simulink library "Contact_Forces_Lib"  (R2019b)
settings: Solver=ode45  StartTime=0.0  StopTime=10.0  RelTol=1e-3  EnableMultiTasking=on
undefined symbols (not defined in the file): b_contact, ball, custom_param_1, custom_param_2, Extr_Data_Ring, k_contact, l_cone, length_cylinder, length_tube, mu_kinetic, mu_static, pen_exponent, pen_full_damp_F, rad_s_cone, radius_cylinder, radius_tube, tube, v_thr, X, Y, Z
libraries: nesl_utility x166, sm_lib x109, $bdroot x65, simulink x14, fl_lib x1
(part 8 of 10)

== system Contact_Forces_Lib/2D/Composite Forces/Box to Box Force/BoxF Corners ==
  Circle to Line C1 AC : $bdroot/2D/Circle to Finite Line Force  circle_rad=boxF_contact_rad  line_depth=boxB_h/2  line_length=boxB_l  force_law=Linear  k_contact=k_contact_box2box  b_contact=b_contact_box2box  pen_full_damp_F=pen_full_damp_F_box2box  pen_exponent=pen_exponent_box2box  custom_param_1=1  custom_param_2=1  friction_law=None  mu_kinetic=mu_kinetic_box2box  mu_static=mu_static_box2box  v_thr=v_thr_box2box  vis_on=off  vis_opc_en=0  vis_len_linBz=vis_len_boxBz  vis_len_linBx=vis_len_boxBx  vis_len_cirFz=vis_len_boxFz  vis_len_cirFx=vis_len_boxFx  vis_clr=vis_clr_box2box  vis_opc=vis_opc_box2box
  Circle to Line C1 BD : $bdroot/2D/Circle to Finite Line Force  circle_rad=boxF_contact_rad  line_depth=boxB_l/2  line_length=boxB_h  force_law=Linear  k_contact=k_contact_box2box  b_contact=b_contact_box2box  pen_full_damp_F=pen_full_damp_F_box2box  pen_exponent=pen_exponent_box2box  custom_param_1=1  custom_param_2=1  friction_law=None  mu_kinetic=mu_kinetic_box2box  mu_static=mu_static_box2box  v_thr=v_thr_box2box  vis_on=off  vis_opc_en=0  vis_len_linBz=vis_len_boxBz  vis_len_linBx=vis_len_boxBx  vis_len_cirFz=vis_len_boxFz  vis_len_cirFx=vis_len_boxFx  vis_clr=vis_clr_box2box  vis_opc=vis_opc_box2box
  Circle to Line C2 AC : $bdroot/2D/Circle to Finite Line Force  circle_rad=boxF_contact_rad  line_depth=boxB_h/2  line_length=boxB_l  force_law=Linear  k_contact=k_contact_box2box  b_contact=b_contact_box2box  pen_full_damp_F=pen_full_damp_F_box2box  pen_exponent=pen_exponent_box2box  custom_param_1=1  custom_param_2=1  friction_law=None  mu_kinetic=mu_kinetic_box2box  mu_static=mu_static_box2box  v_thr=v_thr_box2box  vis_on=off  vis_opc_en=0  vis_len_linBz=vis_len_boxBz  vis_len_linBx=vis_len_boxBx  vis_len_cirFz=vis_len_boxFz  vis_len_cirFx=vis_len_boxFx  vis_clr=vis_clr_box2box  vis_opc=vis_opc_box2box
  Circle to Line C2 BD : $bdroot/2D/Circle to Finite Line Force  circle_rad=boxF_contact_rad  line_depth=boxB_l/2  line_length=boxB_h  force_law=Linear  k_contact=k_contact_box2box  b_contact=b_contact_box2box  pen_full_damp_F=pen_full_damp_F_box2box  pen_exponent=pen_exponent_box2box  custom_param_1=1  custom_param_2=1  friction_law=None  mu_kinetic=mu_kinetic_box2box  mu_static=mu_static_box2box  v_thr=v_thr_box2box  vis_on=off  vis_opc_en=0  vis_len_linBz=vis_len_boxBz  vis_len_linBx=vis_len_boxBx  vis_len_cirFz=vis_len_boxFz  vis_len_cirFx=vis_len_boxFx  vis_clr=vis_clr_box2box  vis_opc=vis_opc_box2box
  Circle to Line C3 AC : $bdroot/2D/Circle to Finite Line Force  circle_rad=boxF_contact_rad  line_depth=boxB_h/2  line_length=boxB_l  force_law=Linear  k_contact=k_contact_box2box  b_contact=b_contact_box2box  pen_full_damp_F=pen_full_damp_F_box2box  pen_exponent=pen_exponent_box2box  custom_param_1=1  custom_param_2=1  friction_law=None  mu_kinetic=mu_kinetic_box2box  mu_static=mu_static_box2box  v_thr=v_thr_box2box  vis_on=off  vis_opc_en=0  vis_len_linBz=vis_len_boxBz  vis_len_linBx=vis_len_boxBx  vis_len_cirFz=vis_len_boxFz  vis_len_cirFx=vis_len_boxFx  vis_clr=vis_clr_box2box  vis_opc=vis_opc_box2box
  Circle to Line C3 BD : $bdroot/2D/Circle to Finite Line Force  circle_rad=boxF_contact_rad  line_depth=boxB_l/2  line_length=boxB_h  force_law=Linear  k_contact=k_contact_box2box  b_contact=b_contact_box2box  pen_full_damp_F=pen_full_damp_F_box2box  pen_exponent=pen_exponent_box2box  custom_param_1=1  custom_param_2=1  friction_law=None  mu_kinetic=mu_kinetic_box2box  mu_static=mu_static_box2box  v_thr=v_thr_box2box  vis_on=off  vis_opc_en=0  vis_len_linBz=vis_len_boxBz  vis_len_linBx=vis_len_boxBx  vis_len_cirFz=vis_len_boxFz  vis_len_cirFx=vis_len_boxFx  vis_clr=vis_clr_box2box  vis_opc=vis_opc_box2box
  Circle to Line C4 AC : $bdroot/2D/Circle to Finite Line Force  circle_rad=boxF_contact_rad  line_depth=boxB_h/2  line_length=boxB_l  force_law=Linear  k_contact=k_contact_box2box  b_contact=b_contact_box2box  pen_full_damp_F=pen_full_damp_F_box2box  pen_exponent=pen_exponent_box2box  custom_param_1=1  custom_param_2=1  friction_law=None  mu_kinetic=mu_kinetic_box2box  mu_static=mu_static_box2box  v_thr=v_thr_box2box  vis_on=off  vis_opc_en=0  vis_len_linBz=vis_len_boxBz  vis_len_linBx=vis_len_boxBx  vis_len_cirFz=vis_len_boxFz  vis_len_cirFx=vis_len_boxFx  vis_clr=vis_clr_box2box  vis_opc=vis_opc_box2box
  Circle to Line C4 BD : $bdroot/2D/Circle to Finite Line Force  circle_rad=boxF_contact_rad  line_depth=boxB_l/2  line_length=boxB_h  force_law=Linear  k_contact=k_contact_box2box  b_contact=b_contact_box2box  pen_full_damp_F=pen_full_damp_F_box2box  pen_exponent=pen_exponent_box2box  custom_param_1=1  custom_param_2=1  friction_law=None  mu_kinetic=mu_kinetic_box2box  mu_static=mu_static_box2box  v_thr=v_thr_box2box  vis_on=off  vis_opc_en=0  vis_len_linBz=vis_len_boxBz  vis_len_linBx=vis_len_boxBx  vis_len_cirFz=vis_len_boxFz  vis_len_cirFx=vis_len_boxFx  vis_clr=vis_clr_box2box  vis_opc=vis_opc_box2box
  Forces : Subsystem
  Transform BD : sm_lib/Frames and Transforms/Rigid Transform  TranslationMethod=None  TranslationStandardOffset=0.1  TranslationLengthUnit=m  TranslationStandardAxis=+Y  TranslationCartesianOffset=[0 0 0]  TranslationROffset=0  TranslationROffsetUnits=m  TranslationZOffset=0  TranslationZOffsetUnits=m  TranslationThetaOffset=0  TranslationThetaOffsetUnits=deg  RotationMethod=StandardAxis  RotationAngleUnits=deg  RotationStandardAxis=+Z  RotationAngle=90  RotationArbitraryAxis=[0 0 1]  FollAlignAxisA=+X  BaseAlignAxisA=+Y  FollAlignAxisB=+Y  BaseAlignAxisB=+Z  RotationSequenceAxes=FollowerAxes  RotationSequence=XYX  RotationSequenceAngles=[0 0 0]  RotationSequenceAnglesUnits=deg  RotationMatrix=[1 0 0; 0 1 0; 0 0 1]
  Transform C1 : sm_lib/Frames and Transforms/Rigid Transform  TranslationMethod=Cartesian  TranslationStandardOffset=0.1  TranslationLengthUnit=m  TranslationStandardAxis=+Y  TranslationCartesianOffset=[-(boxF_h/2-boxF_contact_rad) -(boxF_l/2-boxF_contact_rad) 0]  TranslationROffset=0  TranslationROffsetUnits=m  TranslationZOffset=0  TranslationZOffsetUnits=m  TranslationThetaOffset=0  TranslationThetaOffsetUnits=deg  RotationMethod=None  RotationAngleUnits=deg  RotationStandardAxis=+Z  RotationAngle=0  RotationArbitraryAxis=[0 0 1]  FollAlignAxisA=+X  BaseAlignAxisA=+Y  FollAlignAxisB=+Y  BaseAlignAxisB=+Z  RotationSequenceAxes=FollowerAxes  RotationSequence=XYX  RotationSequenceAngles=[0 0 0]  RotationSequenceAnglesUnits=deg  RotationMatrix=[1 0 0; 0 1 0; 0 0 1]
  Transform C2 : sm_lib/Frames and Transforms/Rigid Transform  TranslationMethod=Cartesian  TranslationStandardOffset=0.1  TranslationLengthUnit=m  TranslationStandardAxis=+Y  TranslationCartesianOffset=[-(boxF_h/2-boxF_contact_rad) (boxF_l/2-boxF_contact_rad) 0]  TranslationROffset=0  TranslationROffsetUnits=m  TranslationZOffset=0  TranslationZOffsetUnits=m  TranslationThetaOffset=0  TranslationThetaOffsetUnits=deg  RotationMethod=None  RotationAngleUnits=deg  RotationStandardAxis=+Z  RotationAngle=0  RotationArbitraryAxis=[0 0 1]  FollAlignAxisA=+X  BaseAlignAxisA=+Y  FollAlignAxisB=+Y  BaseAlignAxisB=+Z  RotationSequenceAxes=FollowerAxes  RotationSequence=XYX  RotationSequenceAngles=[0 0 0]  RotationSequenceAnglesUnits=deg  RotationMatrix=[1 0 0; 0 1 0; 0 0 1]
  Transform C3 : sm_lib/Frames and Transforms/Rigid Transform  TranslationMethod=Cartesian  TranslationStandardOffset=0.1  TranslationLengthUnit=m  TranslationStandardAxis=+Y  TranslationCartesianOffset=[(boxF_h/2-boxF_contact_rad) (boxF_l/2-boxF_contact_rad) 0]  TranslationROffset=0  TranslationROffsetUnits=m  TranslationZOffset=0  TranslationZOffsetUnits=m  TranslationThetaOffset=0  TranslationThetaOffsetUnits=deg  RotationMethod=None  RotationAngleUnits=deg  RotationStandardAxis=+Z  RotationAngle=0  RotationArbitraryAxis=[0 0 1]  FollAlignAxisA=+X  BaseAlignAxisA=+Y  FollAlignAxisB=+Y  BaseAlignAxisB=+Z  RotationSequenceAxes=FollowerAxes  RotationSequence=XYX  RotationSequenceAngles=[0 0 0]  RotationSequenceAnglesUnits=deg  RotationMatrix=[1 0 0; 0 1 0; 0 0 1]
  Transform C4 : sm_lib/Frames and Transforms/Rigid Transform  TranslationMethod=Cartesian  TranslationStandardOffset=0.1  TranslationLengthUnit=m  TranslationStandardAxis=+Y  TranslationCartesianOffset=[(boxF_h/2-boxF_contact_rad) -(boxF_l/2-boxF_contact_rad) 0]  TranslationROffset=0  TranslationROffsetUnits=m  TranslationZOffset=0  TranslationZOffsetUnits=m  TranslationThetaOffset=0  TranslationThetaOffsetUnits=deg  RotationMethod=None  RotationAngleUnits=deg  RotationStandardAxis=+Z  RotationAngle=0  RotationArbitraryAxis=[0 0 1]  FollAlignAxisA=+X  BaseAlignAxisA=+Y  FollAlignAxisB=+Y  BaseAlignAxisB=+Z  RotationSequenceAxes=FollowerAxes  RotationSequence=XYX  RotationSequenceAngles=[0 0 0]  RotationSequenceAnglesUnits=deg  RotationMatrix=[1 0 0; 0 1 0; 0 0 1]
  BoxB : PMIOPort  Side=Left
  BoxF : PMIOPort  Port=2  Side=Right
  wires:
  Circle to Line C4 AC/1 -> Forces/7(4AC)
  Circle to Line C1 BD/1 -> Forces/2(1BD)
  Circle to Line C2 AC/1 -> Forces/3(2AC)
  Circle to Line C3 BD/1 -> Forces/6(3BD)
  Circle to Line C4 BD/1 -> Forces/8(4BD)
  Circle to Line C2 BD/1 -> Forces/4(2BD)
  Circle to Line C3 AC/1 -> Forces/5(3AC)
  Circle to Line C1 AC/1 -> Forces/1(1AC)
  connections:
  Circle to Line C1 BD/RConn1 -- Transform BD/RConn1 -- Circle to Line C3 BD/RConn1 -- Circle to Line C4 BD/RConn1 -- Circle to Line C2 BD/RConn1
  Circle to Line C2 AC/LConn1 -- Circle to Line C2 BD/LConn1 -- Transform C2/RConn1
  Circle to Line C3 AC/LConn1 -- Circle to Line C3 BD/LConn1 -- Transform C3/RConn1
  Transform C3/LConn1 -- Transform C4/LConn1 -- Transform C1/LConn1 -- Transform C2/LConn1 -- BoxF/RConn1
  Circle to Line C4 AC/LConn1 -- Circle to Line C4 BD/LConn1 -- Transform C4/RConn1
  Transform BD/LConn1 -- Circle to Line C1 AC/RConn1 -- Circle to Line C2 AC/RConn1 -- Circle to Line C3 AC/RConn1 -- Circle to Line C4 AC/RConn1 -- BoxB/RConn1
  Circle to Line C1 BD/LConn1 -- Circle to Line C1 AC/LConn1 -- Transform C1/RConn1

== system Contact_Forces_Lib/3D/Prototype/Cone in Ring Force/Enable ==
  z : Inport
  R : Inport  Port=2
  Add1 : Sum  Inputs=+-
  Add3 : Sum  Inputs=+-
  Constant1 : Constant  Value=l_cyl/2+lc
  Constant2 : Constant  Value=l_tube/2
  Constant4 : Constant  Value=l_cyl/2
  Constant5 : Constant  Value=l_tube/2
  Logical Operator : Logic  AllPortsSameDT=off  OutDataTypeStr=boolean
  Product : Product
  Product1 : Product
  Relational Operator1 : RelationalOperator  OutDataTypeStr=boolean  ZeroCross=off  RndMeth=Nearest
  Relational Operator2 : RelationalOperator  Operator=<=  OutDataTypeStr=boolean  ZeroCross=off  RndMeth=Nearest
  Selector : Selector  NumberOfDimensions=2  InputPortWidth=3  IndexOptions=Index vector (dialog),Index vector (dialog)  Indices=3,3  OutputSizes=1,1
  Enable : Outport
  wires:
  Constant5/1 -> Relational Operator1/2
  Add3/1 -> Relational Operator1/1
  Relational Operator1/1 -> Logical Operator/1
  Constant2/1 -> Relational Operator2/2
  z/1 -> Add1/1, Add3/1
  Add1/1 -> Relational Operator2/1
  Relational Operator2/1 -> Logical Operator/2
  Logical Operator/1 -> Enable/1
  R/1 -> Selector/1
  Constant4/1 -> Product/1
  Product/1 -> Add3/2
  Selector/1 -> Product1/1, Product/2  "r33"
  Constant1/1 -> Product1/2
  Product1/1 -> Add1/2

== system Contact_Forces_Lib/3D/Prototype/Cone in Ring Force/If Action Subsystem ==
  Action Port : ActionPort
  Constant : Constant  Value=[0 0 0]  SampleTime=0
  F : Outport
  T : Outport  Port=2
  wires:
  Constant/1 -> T/1, F/1

== system Contact_Forces_Lib/3D/Prototype/Cone in Ring Force/Point of Contact calc ==
  note: Xb = r11*r*cos(th) + r12*r*sin(th) +r13*z + Xc;
      | Yb = r21*r*cos(th) + r22*r*sin(th) +r23*z + Yc;
  R : Inport
  x : Inport  Port=2
  y : Inport  Port=3
  z : Inport  Port=4
  Action Port : ActionPort
  Constant1 : Constant  Value=[0:2*pi/n:2*pi]
  Cross Product : Subsystem
  Demux : Demux  Outputs=3
  Demux1 : Demux  Outputs=3
  Demux2 : Demux  Outputs=3
  Force Calc : Subsystem
  Mux : Mux  Inputs=3
  R1 : InportShadow
  Selector : Selector  NumberOfDimensions=2  InputPortWidth=3  IndexOptions=Index vector (dialog),Index vector (dialog)  Indices=1,[1:3]  OutputSizes=1,1
  Selector1 : Selector  NumberOfDimensions=2  InputPortWidth=3  IndexOptions=Index vector (dialog),Index vector (dialog)  Indices=2,[1:3]  OutputSizes=1,1
  Selector2 : Selector  NumberOfDimensions=2  InputPortWidth=3  IndexOptions=Index vector (dialog),Index vector (dialog)  Indices=3,[1:3]  OutputSizes=1,1
  r calc : Subsystem
  x calc : Subsystem
  y calc : Subsystem
  z calc : Subsystem
  F : Outport
  T : Outport  Port=2
  wires:
  R/1 -> Selector2/1, Selector1/1, Selector/1
  Selector/1 -> Demux/1
  Selector1/1 -> Demux1/1
  Selector2/1 -> Demux2/1
  Demux2/1 -> z calc/1(r31)  "r31"
  Demux2/2 -> z calc/2(r32)  "r32"
  Demux2/3 -> z calc/3(r33)  "r33"
  z/1 -> z calc/4(zc)
  Constant1/1 -> Force Calc/5(th), x calc/5(th), y calc/5(th), z calc/5(th)
  Demux/1 -> x calc/1(r11)
  Demux/2 -> x calc/2(r12)
  Demux/3 -> x calc/3(r13)
  x/1 -> x calc/4(xc)
  z calc/1(z) -> Force Calc/4(z), y calc/6(z), x calc/6(z), r calc/1(z)
  Demux1/1 -> y calc/1(r21)
  Demux1/2 -> y calc/2(r22)
  Demux1/3 -> y calc/3(r23)
  y/1 -> y calc/4(yc)
  x calc/1(x) -> Force Calc/1(x)
  y calc/1(y) -> Force Calc/2(y)
  Force Calc/1(Fx) -> Mux/1
  Force Calc/2(Fy) -> Mux/2
  r calc/1(r) -> Force Calc/3(r), x calc/7(r), y calc/7(r)
  Force Calc/3(Fz) -> Mux/3
  Mux/1 -> Cross Product/2(In2), F/1
  Force Calc/4(pc) -> Cross Product/1(In1)
  Cross Product/1(Out1) -> T/1

== system Contact_Forces_Lib/3D/Prototype/Cylinder In Ring Force/Enable ==
  z : Inport
  R : Inport  Port=2
  Abs : Abs  ZeroCross=off
  Add2 : Sum
  Add3 : Sum  Inputs=+-
  Constant2 : Constant  Value=l_tube/2
  Constant3 : Constant  Value=l_cyl/2
  Constant4 : Constant  Value=l_cyl/2
  Constant5 : Constant  Value=l_tube/2
  Logical Operator : Logic  AllPortsSameDT=off  OutDataTypeStr=boolean
  Product : Product
  Product1 : Product
  Relational Operator : RelationalOperator  OutDataTypeStr=boolean  ZeroCross=off  RndMeth=Nearest
  Relational Operator1 : RelationalOperator  Operator=<=  OutDataTypeStr=boolean  ZeroCross=off  RndMeth=Nearest
  Selector : Selector  NumberOfDimensions=2  InputPortWidth=3  IndexOptions=Index vector (dialog),Index vector (dialog)  Indices=3,3  OutputSizes=1,1
  Enable : Outport
  wires:
  z/1 -> Abs/1
  Logical Operator/1 -> Enable/1
  Constant5/1 -> Relational Operator1/2
  Constant2/1 -> Relational Operator/2
  Relational Operator/1 -> Logical Operator/1
  Abs/1 -> Add3/1, Add2/2
  Relational Operator1/1 -> Logical Operator/2
  Add2/1 -> Relational Operator/1
  Add3/1 -> Relational Operator1/1
  R/1 -> Selector/1
  Selector/1 -> Product1/2, Product/1  "r33"
  Product/1 -> Add3/2
  Constant4/1 -> Product/2
  Product1/1 -> Add2/1
  Constant3/1 -> Product1/1

== system Contact_Forces_Lib/3D/Prototype/Cylinder In Ring Force/If Action Subsystem ==
  Action Port : ActionPort
  Constant : Constant  Value=[0 0 0]  SampleTime=0
  F : Outport
  T : Outport  Port=2
  wires:
  Constant/1 -> T/1, F/1

== system Contact_Forces_Lib/3D/Prototype/Cylinder In Ring Force/Point of Contact calc ==
  note: z = (L/2 - r31*r*cos(th) - r32*r*sin(th) - Zc)/r33;
      | Xb = r11*r*cos(th) + r12*r*sin(th) +r13*z + Xc;
      | Yb = r21*r*cos(th) + r22*r*sin(th) +r23*z + Yc;
  R : Inport
  x : Inport  Port=2
  y : Inport  Port=3
  z : Inport  Port=4
  vz : Inport  Port=5
  Action Port : ActionPort
  Constant1 : Constant  Value=[0:2*pi/n:2*pi]
  Cross Product : Subsystem
  Demux : Demux  Outputs=3
  Demux1 : Demux  Outputs=3
  Demux2 : Demux  Outputs=3
  Divide : Product  Inputs=/*  Multiplication=Matrix(*)
  Force Calc : Subsystem
  Mux : Mux  Inputs=3
  R1 : InportShadow
  Selector : Selector  NumberOfDimensions=2  InputPortWidth=3  IndexOptions=Index vector (dialog),Index vector (dialog)  Indices=1,[1:3]  OutputSizes=1,1
  Selector1 : Selector  NumberOfDimensions=2  InputPortWidth=3  IndexOptions=Index vector (dialog),Index vector (dialog)  Indices=2,[1:3]  OutputSizes=1,1
  Selector2 : Selector  NumberOfDimensions=2  InputPortWidth=3  IndexOptions=Index vector (dialog),Index vector (dialog)  Indices=3,[1:3]  OutputSizes=1,1
  x calc : Subsystem
  y calc : Subsystem
  z calc : Subsystem
  F : Outport
  T : Outport  Port=2
  pen : Outport  Port=3
  wires:
  R/1 -> Selector2/1, Selector1/1, Selector/1
  Selector/1 -> Demux/1
  Selector1/1 -> Demux1/1
  Selector2/1 -> Demux2/1
  Demux2/1 -> z calc/1(r31)  "r31"
  Demux2/2 -> z calc/2(r32)  "r32"
  Demux2/3 -> z calc/3(r33)  "r33"
  z/1 -> z calc/4(zc)
  Constant1/1 -> Force Calc/5(th), y calc/5(th), x calc/5(th), z calc/5(th)
  Demux/1 -> x calc/1(r11)
  Demux/2 -> x calc/2(r12)
  Demux/3 -> x calc/3(r13)
  x/1 -> x calc/4(xc)
  z calc/1(z) -> Force Calc/4(z), y calc/6(z), x calc/6(z)
  Demux1/1 -> y calc/1(r21)
  Demux1/2 -> y calc/2(r22)
  Demux1/3 -> y calc/3(r23)
  y/1 -> y calc/4(yc)
  x calc/1(x) -> Force Calc/1(x)
  y calc/1(y) -> Force Calc/2(y)
  R1/1 -> Divide/1
  Force Calc/1(Fx) -> Mux/1
  Force Calc/2(Fy) -> Mux/2
  Mux/1 -> Divide/2
  Divide/1 -> Cross Product/2(In2), F/1
  Force Calc/3(Fz) -> Mux/3
  Force Calc/4(pc) -> Cross Product/1(In1)
  Cross Product/1(Out1) -> T/1
  vz/1 -> Force Calc/3(v)
  Force Calc/5(maxpen) -> pen/1

== system Contact_Forces_Lib/3D/Sphere in Sphere Force/Ff/Check w or v non zero ==
  w : Inport
  v : Inport  Port=2
  Else : Subsystem  TreatAsAtomicUnit=on
  If : If  NumInputs=2  IfExpression=u1 ~= 0 | u2~=0
  mag v : Subsystem
  mag w : Subsystem
  else v is 0 : Outport
  else uv is 0 : Outport  Port=2
  Use SlipVel : Outport  Port=3
  wires:
  Else/2(vuvect) -> else uv is 0/1
  Else/1(vabs) -> else v is 0/1
  If/2 -> Else/Action
  If/1 -> Use SlipVel/1
  mag w/1(mag) -> If/1
  mag v/1(mag) -> If/2
  v/1 -> mag v/1(vect)
  w/1 -> mag w/1(vect)

== system Contact_Forces_Lib/3D/Sphere in Sphere Force/Ff/SlipVel ==
  w : Inport
  v : Inport  Port=2
  dvect : Inport  Port=3
  Action Port : ActionPort
  Add : Sum
  Add1 : Sum  Inputs=+-
  Add2 : Sum  Inputs=+++
  Cross Product : $bdroot/Math/Cross Product
  Demux : Demux  Outputs=3
  Dot Product : DotProduct  InputSameDT=on  OutDataTypeStr=Inherit: Inherit via internal rule
  Fsphere_rad : Gain  Gain=sphF_rad
  Gain : Gain
  If : If  ShowElse=off
  If Action Subsystem : Subsystem  TreatAsAtomicUnit=on
  Math Function : Math  Operator=square  SaturateOnIntegerOverflow=on
  Math Function1 : Math  Operator=square  SaturateOnIntegerOverflow=on
  Math Function2 : Math  Operator=square  SaturateOnIntegerOverflow=on
  Product : Product
  Sqrt : Sqrt  SaturateOnIntegerOverflow=on
  mag : Subsystem
  vabs : Outport  InitialOutput=0
  vuvect : Outport  Port=2  InitialOutput=0
  wires:
  If Action Subsystem/1(Out1) -> vuvect/1
  If/1 -> If Action Subsystem/Action
  Fsphere_rad/1 -> Cross Product/2
  w/1 -> Cross Product/1
  Cross Product/1 -> Add/1
  v/1 -> Add/2
  dvect/1 -> Gain/1
  Add/1 -> Add1/1, Dot Product/1
  Dot Product/1 -> Product/1
  Product/1 -> Add1/2
  Add1/1 -> Demux/1, mag/1(vect), If Action Subsystem/2(In2)
  Demux/1 -> Math Function/1
  Demux/2 -> Math Function1/1
  Demux/3 -> Math Function2/1
  Math Function/1 -> Add2/1
  Math Function1/1 -> Add2/2
  Math Function2/1 -> Add2/3
  Add2/1 -> Sqrt/1
  Sqrt/1 -> vabs/1
  mag/1(mag) -> If/1, If Action Subsystem/1(In1)
  Gain/1 -> Product/2, Dot Product/2, Fsphere_rad/1

== system Contact_Forces_Lib/3D/Sphere in Sphere Force/Ff/mag ==
  vect : Inport
  Add2 : Sum  Inputs=+++
  Demux : Demux  Outputs=3
  Math Function : Math  Operator=square  SaturateOnIntegerOverflow=on
  Math Function1 : Math  Operator=square  SaturateOnIntegerOverflow=on
  Math Function2 : Math  Operator=square  SaturateOnIntegerOverflow=on
  Sqrt : Sqrt  SaturateOnIntegerOverflow=on
  mag : Outport
  wires:
  Math Function2/1 -> Add2/3
  Demux/3 -> Math Function2/1
  Sqrt/1 -> mag/1
  Math Function1/1 -> Add2/2
  Math Function/1 -> Add2/1
  Add2/1 -> Sqrt/1
  vect/1 -> Demux/1
  Demux/1 -> Math Function/1
  Demux/2 -> Math Function1/1

== system Contact_Forces_Lib/3D/Sphere to Plane Force/Forces/Calculate Penetration ==
  z : Inport
  vz : Inport  Port=2
  Abs : Abs  ZeroCross=off
  Constant : Constant  Value=sphere_rad+plane_depth
  Dead Zone : DeadZone  LowerValue=-inf  UpperValue=0  SaturateOnIntegerOverflow=on
  Gain2 : Gain  Gain=-1
  Product : Product
  Sign vx : Signum  ZeroCross=off
  Sign x : Signum  ZeroCross=off
  Sum : Sum  Inputs=+-
  Pos Sign : Outport
  Pen : Outport  Port=2
  Pen Vel : Outport  Port=3
  Vel Sign : Outport  Port=4
  wires:
  z/1 -> Sign x/1, Abs/1
  vz/1 -> Product/2, Sign vx/1
  Constant/1 -> Sum/1
  Sum/1 -> Dead Zone/1
  Abs/1 -> Sum/2
  Sign x/1 -> Pos Sign/1, Product/1
  Sign vx/1 -> Vel Sign/1
  Product/1 -> Gain2/1
  Dead Zone/1 -> Pen/1
  Gain2/1 -> Pen Vel/1

== system Contact_Forces_Lib/3D/Sphere to Plane Force/Forces/Ff ==
  Fn : Inport
  R : Inport  Port=2
  zSign : Inport  Port=3
  wx : Inport  Port=4
  wy : Inport  Port=5
  vx : Inport  Port=6
  vy : Inport  Port=7
  Cross Product : $bdroot/Math/Cross Product
  Friction Law : $bdroot/Friction Law  OverrideUsingVariant=Stick_Slip_C
  Fx1 : Constant  Value=0
  Fx2 : Constant  Value=[0 0 -sphere_rad]
  Gain : Gain  Gain=-1
  Mux1 : Mux  Inputs=3
  Product1 : Product  Inputs=/*  Multiplication=Matrix(*)
  Product2 : Product  Inputs=/*  Multiplication=Matrix(*)
  Product{3..7} (5 alike) : Product
  Selector : Selector  InputPortWidth=3  IndexOptions=Index vector (dialog)  Indices=3  OutputSizes=1
  SlipVel : Subsystem
  Trigonometric Function : Trigonometry
  Trigonometric Function1 : Trigonometry  Operator=cos
  zSign1 : InportShadow  Port=3
  Ff Sph : Outport
  T Sph : Outport  Port=2
  Ff Pla : Outport  Port=3
  wires:
  Fn/1 -> Selector/1
  Gain/1 -> Ff Pla/1
  SlipVel/2(alpha) -> Trigonometric Function/1, Trigonometric Function1/1
  Trigonometric Function1/1 -> Product3/2
  SlipVel/1(vabs) -> Friction Law/2
  Selector/1 -> Friction Law/1
  Friction Law/1 -> Product3/1, Product4/1
  Product4/1 -> Mux1/2
  Product3/1 -> Mux1/1
  Fx1/1 -> Mux1/3
  Trigonometric Function/1 -> Product4/2
  vx/1 -> Product6/1
  wx/1 -> SlipVel/1(wx)
  wy/1 -> SlipVel/2(wy)
  vy/1 -> Product5/2
  Product2/1 -> T Sph/1
  Mux1/1 -> Gain/1, Cross Product/2, Product1/2
  Product1/1 -> Ff Sph/1
  Cross Product/1 -> Product2/2
  R/1 -> Product1/1, Product2/1
  Fx2/1 -> Product7/1
  Product5/1 -> SlipVel/4(vy)
  zSign/1 -> Product5/1, Product6/2
  Product6/1 -> SlipVel/3(vx)
  zSign1/1 -> Product7/2
  Product7/1 -> Cross Product/1

== system Contact_Forces_Lib/3D/Sphere to Plane Force/Forces/Fn ==
  R : Inport
  SprF : Inport  Port=2
  DamF : Inport  Port=3
  Fx : Constant  Value=0
  Gain : Gain  Gain=-1
  Mux : Mux  Inputs=3
  Product2 : Product  Inputs=/*  Multiplication=Matrix(*)
  Sum : Sum
  Fn : Outport
  FnF : Outport  Port=2
  FnB : Outport  Port=3
  wires:
  Mux/1 -> Gain/1, Product2/2
  Product2/1 -> FnF/1
  Gain/1 -> FnB/1
  R/1 -> Product2/1
  Fx/1 -> Mux/1, Mux/2
  Sum/1 -> Fn/1, Mux/3
  DamF/1 -> Sum/2
  SprF/1 -> Sum/1

== system Contact_Forces_Lib/3D/Sphere to Plane Force Enabled/Forces/Calculate Penetration ==
  z : Inport
  vz : Inport  Port=2
  Abs : Abs  ZeroCross=off
  Constant : Constant  Value=sphere_rad+plane_depth
  Dead Zone : DeadZone  LowerValue=-inf  UpperValue=0  SaturateOnIntegerOverflow=on
  Gain2 : Gain  Gain=-1
  Product : Product
  Sign vx : Signum  ZeroCross=off
  Sign x : Signum  ZeroCross=off
  Sum : Sum  Inputs=+-
  Pos Sign : Outport
  Pen : Outport  Port=2
  Pen Vel : Outport  Port=3
  Vel Sign : Outport  Port=4
  wires:
  Gain2/1 -> Pen Vel/1
  Dead Zone/1 -> Pen/1
  Product/1 -> Gain2/1
  Sign vx/1 -> Vel Sign/1
  Sign x/1 -> Product/1, Pos Sign/1
  Abs/1 -> Sum/2
  Sum/1 -> Dead Zone/1
  Constant/1 -> Sum/1
  vz/1 -> Sign vx/1, Product/2
  z/1 -> Abs/1, Sign x/1

== system Contact_Forces_Lib/3D/Sphere to Plane Force Enabled/Forces/Ff ==
  Fn : Inport
  R : Inport  Port=2
  zSign : Inport  Port=3
  wx : Inport  Port=4
  wy : Inport  Port=5
  vx : Inport  Port=6
  vy : Inport  Port=7
  Cross Product : $bdroot/Math/Cross Product
  Friction Law : $bdroot/Friction Law  OverrideUsingVariant=Stick_Slip_C
  Fx1 : Constant  Value=0
  Fx2 : Constant  Value=[0 0 -sphere_rad]
  Gain : Gain  Gain=-1
  Mux1 : Mux  Inputs=3
  Product1 : Product  Inputs=/*  Multiplication=Matrix(*)
  Product2 : Product  Inputs=/*  Multiplication=Matrix(*)
  Product{3..7} (5 alike) : Product
  Selector : Selector  InputPortWidth=3  IndexOptions=Index vector (dialog)  Indices=3  OutputSizes=1
  SlipVel : Subsystem
  Trigonometric Function : Trigonometry
  Trigonometric Function1 : Trigonometry  Operator=cos
  zSign1 : InportShadow  Port=3
  Ff Sph : Outport
  T Sph : Outport  Port=2
  Ff Pla : Outport  Port=3
  wires:
  Product7/1 -> Cross Product/1
  zSign1/1 -> Product7/2
  Product6/1 -> SlipVel/3(vx)
  zSign/1 -> Product6/2, Product5/1
  Product5/1 -> SlipVel/4(vy)
  Fx2/1 -> Product7/1
  R/1 -> Product2/1, Product1/1
  Cross Product/1 -> Product2/2
  Product1/1 -> Ff Sph/1
  Mux1/1 -> Product1/2, Cross Product/2, Gain/1
  Product2/1 -> T Sph/1
  vy/1 -> Product5/2
  wy/1 -> SlipVel/2(wy)
  wx/1 -> SlipVel/1(wx)
  vx/1 -> Product6/1
  Trigonometric Function/1 -> Product4/2
  Fx1/1 -> Mux1/3
  Product3/1 -> Mux1/1
  Product4/1 -> Mux1/2
  Friction Law/1 -> Product4/1, Product3/1
  Selector/1 -> Friction Law/1
  SlipVel/1(vabs) -> Friction Law/2
  Trigonometric Function1/1 -> Product3/2
  SlipVel/2(alpha) -> Trigonometric Function1/1, Trigonometric Function/1
  Gain/1 -> Ff Pla/1
  Fn/1 -> Selector/1

== system Contact_Forces_Lib/3D/Sphere to Plane Force Enabled/Forces/Fn ==
  R : Inport
  SprF : Inport  Port=2
  DamF : Inport  Port=3
  Fx : Constant  Value=0
  Gain : Gain  Gain=-1
  Mux : Mux  Inputs=3
  Product2 : Product  Inputs=/*  Multiplication=Matrix(*)
  Sum : Sum
  Fn : Outport
  FnF : Outport  Port=2
  FnB : Outport  Port=3
  wires:
  SprF/1 -> Sum/1
  DamF/1 -> Sum/2
  Sum/1 -> Mux/3, Fn/1
  Fx/1 -> Mux/2, Mux/1
  R/1 -> Product2/1
  Gain/1 -> FnB/1
  Product2/1 -> FnF/1
  Mux/1 -> Product2/2, Gain/1

== system Contact_Forces_Lib/3D/Sphere to Sphere Force/Ff/Check w or v non zero ==
  w : Inport
  v : Inport  Port=2
  Else : Subsystem  TreatAsAtomicUnit=on
  If : If  NumInputs=2  IfExpression=u1 ~= 0 | u2~=0
  mag v : Subsystem
  mag w : Subsystem
  else v is 0 : Outport
  else uv is 0 : Outport  Port=2
  Use SlipVel : Outport  Port=3
  wires:
  w/1 -> mag w/1(vect)
  v/1 -> mag v/1(vect)
  mag v/1(mag) -> If/2
  mag w/1(mag) -> If/1
  If/1 -> Use SlipVel/1
  If/2 -> Else/Action
  Else/1(vabs) -> else v is 0/1
  Else/2(vuvect) -> else uv is 0/1

== system Contact_Forces_Lib/3D/Sphere to Sphere Force/Ff/SlipVel ==
  w : Inport
  v : Inport  Port=2
  dvect : Inport  Port=3
  Action Port : ActionPort
  Add : Sum
  Add1 : Sum  Inputs=+-
  Add2 : Sum  Inputs=+++
  Cross Product : $bdroot/Math/Cross Product
  Demux : Demux  Outputs=3
  Dot Product : DotProduct  InputSameDT=on  OutDataTypeStr=Inherit: Inherit via internal rule
  Fsphere_rad : Gain  Gain=sphF_rad
  Gain : Gain  Gain=-1
  If : If  ShowElse=off
  If Action Subsystem : Subsystem  TreatAsAtomicUnit=on
  Math Function : Math  Operator=square  SaturateOnIntegerOverflow=on
  Math Function1 : Math  Operator=square  SaturateOnIntegerOverflow=on
  Math Function2 : Math  Operator=square  SaturateOnIntegerOverflow=on
  Product : Product
  Sqrt : Sqrt  SaturateOnIntegerOverflow=on
  mag : Subsystem
  vabs : Outport  InitialOutput=0
  vuvect : Outport  Port=2  InitialOutput=0
  wires:
  mag/1(mag) -> If Action Subsystem/1(In1), If/1
  Sqrt/1 -> vabs/1
  Add2/1 -> Sqrt/1
  Math Function2/1 -> Add2/3
  Math Function1/1 -> Add2/2
  Math Function/1 -> Add2/1
  Demux/3 -> Math Function2/1
  Demux/2 -> Math Function1/1
  Demux/1 -> Math Function/1
  Add1/1 -> If Action Subsystem/2(In2), mag/1(vect), Demux/1
  Product/1 -> Add1/2
  Dot Product/1 -> Product/1
  Add/1 -> Dot Product/1, Add1/1
  Gain/1 -> Dot Product/2, Product/2, Fsphere_rad/1
  v/1 -> Add/2
  Cross Product/1 -> Add/1
  dvect/1 -> Gain/1
  w/1 -> Cross Product/1
  Fsphere_rad/1 -> Cross Product/2
  If/1 -> If Action Subsystem/Action
  If Action Subsystem/1(Out1) -> vuvect/1

== system Contact_Forces_Lib/3D/Sphere to Sphere Force/Ff/mag ==
  vect : Inport
  Add2 : Sum  Inputs=+++
  Demux : Demux  Outputs=3
  Math Function : Math  Operator=square  SaturateOnIntegerOverflow=on
  Math Function1 : Math  Operator=square  SaturateOnIntegerOverflow=on
  Math Function2 : Math  Operator=square  SaturateOnIntegerOverflow=on
  Sqrt : Sqrt  SaturateOnIntegerOverflow=on
  mag : Outport
  wires:
  Demux/2 -> Math Function1/1
  Demux/1 -> Math Function/1
  vect/1 -> Demux/1
  Add2/1 -> Sqrt/1
  Math Function/1 -> Add2/1
  Math Function1/1 -> Add2/2
  Sqrt/1 -> mag/1
  Demux/3 -> Math Function2/1
  Math Function2/1 -> Add2/3

== system Contact_Forces_Lib/3D/Sphere to Tube Force/Check Active/Check Active Range ==
  azm : Inport
  " Upper Bound" : simulink/Logic and Bit Operations/Compare To Constant  relop=<=  const=active_angle(2)*pi/180  OutDataTypeStr=boolean  ZeroCross=off
  Logical Operator : Logic  AllPortsSameDT=off  OutDataTypeStr=boolean
  Lower Bound : simulink/Logic and Bit Operations/Compare To Constant  relop=>=  const=active_angle(1)*pi/180  OutDataTypeStr=boolean  ZeroCross=off
  En : Outport
  wires:
  azm/1 -> " Upper Bound"/1, Lower Bound/1
  " Upper Bound"/1 -> Logical Operator/1
  Lower Bound/1 -> Logical Operator/2
  Logical Operator/1 -> En/1

== system Contact_Forces_Lib/3D/Sphere to Tube Force/Check Active/In Tube ==
  z : Inport
  Abs1 : Abs  ZeroCross=off
  Activation limit for contact force : Constant  Value=l_tube/2
  Sum : Sum  Inputs=+-
  En : Outport
  wires:
  Abs1/1 -> Sum/2
  z/1 -> Abs1/1
  Activation limit for contact force/1 -> Sum/1
  Sum/1 -> En/1

== system Contact_Forces_Lib/3D/Sphere to Tube Force/Forces/Calculate Penetration ==
  note: Calculates CirF frame to midpoint of ring wall.
      | Absolute value makes it valid for inside or outside contact.
      | Noting the sign allows us to apply the force correctly
  rad : Inport
  vrad : Inport  Port=2
  Abs : Abs  ZeroCross=off
  Constant : Constant  Value=radius_sphere+d_tube/2
  Dead Zone : DeadZone  LowerValue=-inf  UpperValue=0  SaturateOnIntegerOverflow=on
  Product : Product
  Sign : Signum  ZeroCross=off
  Sum : Sum  Inputs=+-
  Sum1 : Sum  Inputs=+-
  radius ring : Constant  Value=radius_tube
  sign : Outport
  Pen : Outport  Port=2
  Pen Vel : Outport  Port=3
  wires:
  radius ring/1 -> Sum1/1
  Sum1/1 -> Sign/1, Abs/1
  rad/1 -> Sum1/2
  Abs/1 -> Sum/2
  Sign/1 -> Product/1, sign/1
  Product/1 -> Pen Vel/1
  vrad/1 -> Product/2
  Sum/1 -> Dead Zone/1
  Constant/1 -> Sum/1
  Dead Zone/1 -> Pen/1

== system Contact_Forces_Lib/3D/Sphere to Tube Force/Forces/Ff ==
  R : Inport
  azm : Inport  Port=2
  vazm : Inport  Port=3
  wzf : Inport  Port=4
  Fn : Inport  Port=5
  Pen : Inport  Port=6
  rad : Inport  Port=7
  vzf : Inport  Port=8
  wxf : Inport  Port=9
  wyf : Inport  Port=10
  Friction Law : $bdroot/Friction Law  OverrideUsingVariant=Stick_Slip_C
  Resolve Ff : Subsystem
  vTan : Subsystem
  FxSphF : Outport
  FySohF : Outport  Port=2
  FzSphF : Outport  Port=3
  FxTubB : Outport  Port=4
  FyTubB : Outport  Port=5
  FzTubB : Outport  Port=6
  TSphF : Outport  Port=7
  TTubB : Outport  Port=8
  Ff : Outport  Port=9
  wires:
  Resolve Ff/7(FzTubB) -> FzTubB/1
  Resolve Ff/3(FzSphF) -> FzSphF/1
  vTan/2(alpha) -> Resolve Ff/5(alpha)
  vzf/1 -> vTan/6(vzf)
  vTan/1(vabs) -> Friction Law/2
  R/1 -> Resolve Ff/2(R)
  Pen/1 -> vTan/3(Pen)
  Fn/1 -> vTan/1(Fn), Resolve Ff/1(Fn), Friction Law/1
  rad/1 -> vTan/2(rad)
  vazm/1 -> vTan/4(vazm)
  wzf/1 -> vTan/5(wzf)
  Friction Law/1 -> Resolve Ff/3(Ff), Ff/1
  Resolve Ff/1(FxSphF) -> FxSphF/1
  Resolve Ff/2(FySphF) -> FySohF/1
  Resolve Ff/5(FxSphB) -> FxTubB/1
  Resolve Ff/6(FyTubB) -> FyTubB/1
  Resolve Ff/4(TSphF) -> TSphF/1
  Resolve Ff/8(TTubB) -> TTubB/1
  wxf/1 -> vTan/7(wxf)
  wyf/1 -> vTan/8(wyf)
  azm/1 -> vTan/9(azm), Resolve Ff/4(azm)

== system Contact_Forces_Lib/3D/Sphere to Tube Force/Forces/Fn ==
  note: Resolve Normal Force in
      | Tube B reference frame
  note: Resolve Normal Force in
      | Sphere F reference frame
  Fn : Inport
  z : Inport  Port=2
  R : Inport  Port=3
  azm : Inport  Port=4
  Fn in SphF : Subsystem
  Fn in TubB : Subsystem
  Gain : Gain  Gain=-1
  Product : Product
  Product1 : Product
  FxSphF : Outport
  FySphF : Outport  Port=2
  FZSphF : Outport  Port=3
  FxTubB : Outport  Port=4
  FyTubB : Outport  Port=5
  TxTubB : Outport  Port=6
  TyTubB : Outport  Port=7
  wires:
  Product1/1 -> TxTubB/1
  Product/1 -> TyTubB/1
  Gain/1 -> Product1/2
  z/1 -> Product/1, Product1/1
  Fn in SphF/1(FySphF) -> FySphF/1
  Fn in TubB/1(FxTubB) -> FxTubB/1, Product/2, Fn in SphF/2(FxTubB)
  Fn in TubB/2(FyTubB) -> Gain/1, FyTubB/1, Fn in SphF/3(FyTubB)
  Fn/1 -> Fn in TubB/1(Fn)
  azm/1 -> Fn in TubB/2(azm)
  R/1 -> Fn in SphF/1(R)
  Fn in SphF/2(FxSphF) -> FxSphF/1
  Fn in SphF/3(FzSphF) -> FZSphF/1

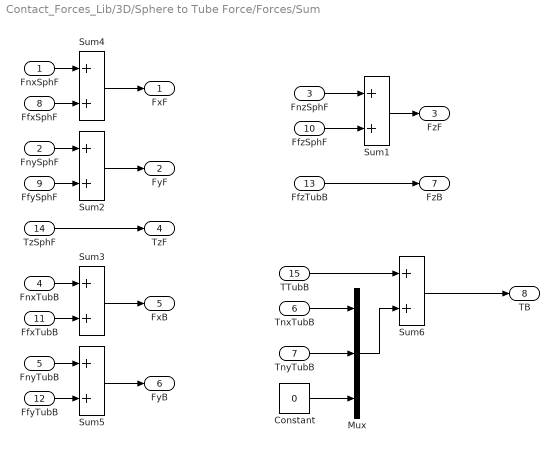
== system Contact_Forces_Lib/3D/Sphere to Tube Force/Forces/Sum ==
  FnxSphF : Inport
  FnySphF : Inport  Port=2
  FnzSphF : Inport  Port=3
  FnxTubB : Inport  Port=4
  FnyTubB : Inport  Port=5
  TnxTubB : Inport  Port=6
  TnyTubB : Inport  Port=7
  FfxSphF : Inport  Port=8
  FfySphF : Inport  Port=9
  FfzSphF : Inport  Port=10
  FfxTubB : Inport  Port=11
  FfyTubB : Inport  Port=12
  FfzTubB : Inport  Port=13
  TzSphF : Inport  Port=14
  TTubB : Inport  Port=15
  Constant : Constant  Value=0
  Mux : Mux  Inputs=3
  Sum{1..6} (6 alike) : Sum
  FxF : Outport
  FyF : Outport  Port=2
  FzF : Outport  Port=3
  TzF : Outport  Port=4
  FxB : Outport  Port=5
  FyB : Outport  Port=6
  FzB : Outport  Port=7
  TB : Outport  Port=8
  wires:
  Constant/1 -> Mux/3
  TnyTubB/1 -> Mux/2
  TnxTubB/1 -> Mux/1
  Mux/1 -> Sum6/2
  TTubB/1 -> Sum6/1
  TzSphF/1 -> TzF/1
  FfyTubB/1 -> Sum5/2
  FfxTubB/1 -> Sum3/2
  FfySphF/1 -> Sum2/2
  FfxSphF/1 -> Sum4/2
  Sum5/1 -> FyB/1
  Sum3/1 -> FxB/1
  Sum2/1 -> FyF/1
  Sum4/1 -> FxF/1
  FnyTubB/1 -> Sum5/1
  FnxTubB/1 -> Sum3/1
  FnySphF/1 -> Sum2/1
  FnxSphF/1 -> Sum4/1
  Sum1/1 -> FzF/1
  FnzSphF/1 -> Sum1/1
  FfzSphF/1 -> Sum1/2
  FfzTubB/1 -> FzB/1
  Sum6/1 -> TB/1

== system Contact_Forces_Lib/3D/Sphere to Tube Force/Sensing/rad_azm_cal ==
  X : Inport
  Y : Inport  Port=2
  Xdot : Inport  Port=3
  Ydot : Inport  Port=4
  Demux : Demux
  If centers are not colocated : If  IfExpression=(u1 > 0)
  Math Function : Math  Operator=square  SaturateOnIntegerOverflow=on
  Math Function1 : Math  Operator=square  SaturateOnIntegerOverflow=on
  Merge : Merge  InitialOutput=0  InputPortOffsets=0
  Sum : Sum  Inputs=|++
  rad_0 : Subsystem
  rad_azm_cal : Subsystem
  rad : Outport
  azm : Outport  Port=2
  radv : Outport  Port=3
  azmv : Outport  Port=4
  wires:
  Merge/1 -> Demux/1
  If centers are not colocated/1 -> rad_azm_cal/Action
  If centers are not colocated/2 -> rad_0/Action
  Demux/2 -> azm/1
  rad_0/1(F) -> Merge/1
  Demux/4 -> azmv/1
  Demux/1 -> rad/1
  Demux/3 -> radv/1
  Xdot/1 -> rad_azm_cal/3(Xdot)
  X/1 -> Math Function/1, rad_azm_cal/1(X)
  Ydot/1 -> rad_azm_cal/4(Ydot)
  Y/1 -> Math Function1/1, rad_azm_cal/2(Y)
  rad_azm_cal/1(F) -> Merge/2
  Math Function1/1 -> Sum/2
  Math Function/1 -> Sum/1
  Sum/1 -> If centers are not colocated/1

== system Contact_Forces_Lib/Friction Utilities/Utilities/Product/FcConst ==
  PS Product : fl_lib/Physical Signals/Functions/PS Product
      settings: SourceProductName=Simscape
  PS-Simulink Converter2 : nesl_utility/PS-Simulink Converter  PhysicalDomain=network_engine_domain  SubClassName=ps_output  LeftPortType=input  RightPortType=output  PseudoPeriodic=off  Frequencies=[]  Unit=1  AffineConversion=off
  Terminator : Terminator
  Fc : PMIOPort  Side=Right
  v : PMIOPort  Port=2  Side=Right
  wires:
  PS-Simulink Converter2/1 -> Terminator/1
  connections:
  PS Product/LConn1 -- v/RConn1
  PS Product/LConn2 -- Fc/RConn1
  PS-Simulink Converter2/LConn1 -- PS Product/RConn1

== system Contact_Forces_Lib/Friction Utilities/Utilities/Product/FcVect ==
  PS-Simulink Converter1 : nesl_utility/PS-Simulink Converter  PhysicalDomain=network_engine_domain  SubClassName=ps_output  LeftPortType=input  RightPortType=output  PseudoPeriodic=off  Frequencies=[]  Unit=1  AffineConversion=off
  PS-Simulink Converter2 : nesl_utility/PS-Simulink Converter  PhysicalDomain=network_engine_domain  SubClassName=ps_output  LeftPortType=input  RightPortType=output  PseudoPeriodic=off  Frequencies=[]  Unit=1  AffineConversion=off
  Terminator : Terminator
  Terminator1 : Terminator
  Fc : PMIOPort  Side=Right
  v : PMIOPort  Port=2  Side=Right
  wires:
  PS-Simulink Converter1/1 -> Terminator1/1
  PS-Simulink Converter2/1 -> Terminator/1
  connections:
  PS-Simulink Converter1/LConn1 -- Fc/RConn1
  PS-Simulink Converter2/LConn1 -- v/RConn1

== system Contact_Forces_Lib/2D/Circle to Circle Force/Ff/Resolve Ff/Ff in CirB ==
  Ff : Inport
  azm : Inport  Port=2
  Divide1 : Product  Inputs=**
  Divide2 : Product  Inputs=**
  Gain3 : Gain  Gain=-1
  cos : Trigonometry
  deg2rad : Gain  Gain=pi/180
  sin : Trigonometry  Operator=cos
  FxCirB : Outport
  FyCirB : Outport  Port=2
  wires:
  Gain3/1 -> Divide1/2
  Ff/1 -> Divide1/1, Divide2/1
  Divide1/1 -> FxCirB/1
  deg2rad/1 -> cos/1, sin/1
  sin/1 -> Divide2/2
  cos/1 -> Gain3/1
  Divide2/1 -> FyCirB/1  "Fy Cir"
  azm/1 -> deg2rad/1

== system Contact_Forces_Lib/2D/Circle to Circle Force/Ff/Resolve Ff/Ff in CirF ==
  R : Inport
  FxCirB : Inport  Port=2
  FyCirB : Inport  Port=3
  Demux : Demux  Outputs=2
  Divide3 : Product  Inputs=**  Multiplication=Matrix(*)
  Gain1 : Gain  Gain=-1
  Mux1 : Mux  Inputs=2
  FyCirF : Outport
  FxCirF : Outport  Port=2
  wires:
  FxCirB/1 -> Mux1/2
  FyCirB/1 -> Mux1/1
  Demux/2 -> FxCirF/1
  Demux/1 -> FyCirF/1
  Gain1/1 -> Demux/1
  Mux1/1 -> Divide3/2
  Divide3/1 -> Gain1/1
  R/1 -> Divide3/1

== system Contact_Forces_Lib/2D/Circle to Circle Force/Ff/Resolve Ff/Tz ==
  Ff : Inport
  Base Radius : Constant  Value=cirB_rad
  Divide4 : Product  Inputs=**
  Divide5 : Product  Inputs=**
  Follower Radius : Constant  Value=cirF_rad
  Gain2 : Gain
  TzB : Outport
  TzF : Outport  Port=2
  wires:
  Ff/1 -> Divide4/2, Gain2/1
  Gain2/1 -> Divide5/1
  Divide4/1 -> TzF/1
  Follower Radius/1 -> Divide4/1
  Divide5/1 -> TzB/1
  Base Radius/1 -> Divide5/2

== system Contact_Forces_Lib/2D/Circle to Circle Force Enabled/Ff/Resolve Ff/Ff in CirB ==
  Ff : Inport
  azm : Inport  Port=2
  Divide1 : Product  Inputs=**
  Divide2 : Product  Inputs=**
  Gain3 : Gain  Gain=-1
  cos : Trigonometry
  deg2rad : Gain  Gain=pi/180
  sin : Trigonometry  Operator=cos
  FxCirB : Outport
  FyCirB : Outport  Port=2
  wires:
  azm/1 -> deg2rad/1
  Divide2/1 -> FyCirB/1  "Fy Cir"
  cos/1 -> Gain3/1
  sin/1 -> Divide2/2
  deg2rad/1 -> sin/1, cos/1
  Divide1/1 -> FxCirB/1
  Ff/1 -> Divide2/1, Divide1/1
  Gain3/1 -> Divide1/2

== system Contact_Forces_Lib/2D/Circle to Circle Force Enabled/Ff/Resolve Ff/Ff in CirF ==
  R : Inport
  FxCirB : Inport  Port=2
  FyCirB : Inport  Port=3
  Demux : Demux  Outputs=2
  Divide3 : Product  Inputs=**  Multiplication=Matrix(*)
  Gain1 : Gain  Gain=-1
  Mux1 : Mux  Inputs=2
  FyCirF : Outport
  FxCirF : Outport  Port=2
  wires:
  R/1 -> Divide3/1
  Divide3/1 -> Gain1/1
  Mux1/1 -> Divide3/2
  Gain1/1 -> Demux/1
  Demux/1 -> FyCirF/1
  Demux/2 -> FxCirF/1
  FyCirB/1 -> Mux1/1
  FxCirB/1 -> Mux1/2

== system Contact_Forces_Lib/2D/Circle to Circle Force Enabled/Ff/Resolve Ff/Tz ==
  Ff : Inport
  Base Radius : Constant  Value=cirB_rad
  Divide4 : Product  Inputs=**
  Divide5 : Product  Inputs=**
  Follower Radius : Constant  Value=cirF_rad
  Gain2 : Gain
  TzB : Outport
  TzF : Outport  Port=2
  wires:
  Base Radius/1 -> Divide5/2
  Divide5/1 -> TzB/1
  Follower Radius/1 -> Divide4/1
  Divide4/1 -> TzF/1
  Gain2/1 -> Divide5/1
  Ff/1 -> Gain2/1, Divide4/2

== system Contact_Forces_Lib/2D/Circle to Finite Line Force/Forces/Resolve Forces/FnCir ==
  note: Calculate circle Normal Force in circle reference frame
  Unit Vector : Inport
  Fn : Inport  Port=2
  Demux1 : Demux  Outputs=2
  Divide1 : Product  Inputs=**
  FxCir : Outport
  FyCir : Outport  Port=2
  wires:
  Unit Vector/1 -> Divide1/2
  Divide1/1 -> Demux1/1
  Fn/1 -> Divide1/1
  Demux1/2 -> FyCir/1  "Fy Cir"
  Demux1/1 -> FxCir/1  "Fx Cir"

== system Contact_Forces_Lib/2D/Circle to Finite Line Force/Forces/Resolve Forces/FnLin ==
  note: Normal Force is calculated in line reference frame,
      | and acts along x-axis only.
  Fn : Inport
  Constant : Constant  Value=0
  Constant1 : Constant  Value=0
  Sum : Sum
  FxLin : Outport
  FyLin : Outport  Port=2
  wires:
  Constant1/1 -> Sum/1
  Sum/1 -> FxLin/1
  Fn/1 -> Sum/2  "Fx Lin"
  Constant/1 -> FyLin/1  "Fy Lin"

== system Contact_Forces_Lib/2D/Circle to Finite Line Force/Forces/Resolve Forces/Friction ==
  Unit Vector : Inport
  Fn : Inport  Port=2
  X Sep : Inport  Port=3
  vLin : Inport  Port=4
  wz : Inport  Port=5
  Components : Gain  Gain=[1 -1]
  Demux : Demux  Outputs=2
  Friction Law : $bdroot/Friction Law  OverrideUsingVariant=None
  Line Ref h : Gain  Gain=line_depth
  Product1 : Product
  Product2 : Product
  Product3 : Product
  Radius : Gain  Gain=-circle_rad
  Sign : Signum
  Sum : Sum  Inputs=-+
  VCirPt : Subsystem
  FxCir : Outport
  FyCir : Outport  Port=2
  FyLin : Outport  Port=3
  TzLin : Outport  Port=4
  TzCir : Outport  Port=5
  Ff : Outport  Port=6
  wires:
  Sign/1 -> Product3/2, Product1/2
  X Sep/1 -> VCirPt/2(X sep), Sign/1
  Product2/1 -> Demux/1
  Radius/1 -> TzCir/1
  Line Ref h/1 -> TzLin/1
  Fn/1 -> Friction Law/1
  Sum/1 -> Friction Law/2
  Unit Vector/1 -> Components/1
  wz/1 -> VCirPt/1(wz)
  Demux/2 -> FxCir/1  "FxCir"
  VCirPt/1(vCir) -> Sum/2
  vLin/1 -> Sum/1
  Demux/1 -> FyCir/1  "FyCir"
  Friction Law/1 -> Product1/1, Radius/1, Ff/1, Product2/2, Line Ref h/1  "Ff"
  Product1/1 -> FyLin/1
  Components/1 -> Product3/1
  Product3/1 -> Product2/1

== system Contact_Forces_Lib/2D/Circle to Finite Line Force Enabled/Forces/Resolve Forces/FnCir ==
  note: Calculate circle Normal Force in circle reference frame
  Unit Vector : Inport
  Fn : Inport  Port=2
  Demux1 : Demux  Outputs=2
  Divide1 : Product  Inputs=**
  FxCir : Outport
  FyCir : Outport  Port=2
  wires:
  Demux1/1 -> FxCir/1  "Fx Cir"
  Demux1/2 -> FyCir/1  "Fy Cir"
  Fn/1 -> Divide1/1
  Divide1/1 -> Demux1/1
  Unit Vector/1 -> Divide1/2

== system Contact_Forces_Lib/2D/Circle to Finite Line Force Enabled/Forces/Resolve Forces/FnLin ==
  note: Normal Force is calculated in line reference frame,
      | and acts along x-axis only.
  Fn : Inport
  Constant : Constant  Value=0
  Constant1 : Constant  Value=0
  Sum : Sum
  FxLin : Outport
  FyLin : Outport  Port=2
  wires:
  Constant/1 -> FyLin/1  "Fy Lin"
  Fn/1 -> Sum/2  "Fx Lin"
  Sum/1 -> FxLin/1
  Constant1/1 -> Sum/1

== system Contact_Forces_Lib/2D/Circle to Finite Line Force Enabled/Forces/Resolve Forces/Friction ==
  Unit Vector : Inport
  Fn : Inport  Port=2
  X Sep : Inport  Port=3
  vLin : Inport  Port=4
  wz : Inport  Port=5
  Components : Gain  Gain=[1 -1]
  Demux : Demux  Outputs=2
  Friction Law : $bdroot/Friction Law  OverrideUsingVariant=None
  Line Ref h : Gain  Gain=line_depth
  Product1 : Product
  Product2 : Product
  Product3 : Product
  Radius : Gain  Gain=-circle_rad
  Sign : Signum
  Sum : Sum  Inputs=-+
  VCirPt : Subsystem
  FxCir : Outport
  FyCir : Outport  Port=2
  FyLin : Outport  Port=3
  TzLin : Outport  Port=4
  TzCir : Outport  Port=5
  Ff : Outport  Port=6
  wires:
  Product3/1 -> Product2/1
  Components/1 -> Product3/1
  Product1/1 -> FyLin/1
  Friction Law/1 -> Line Ref h/1, Product2/2, Ff/1, Radius/1, Product1/1  "Ff"
  Demux/1 -> FyCir/1  "FyCir"
  vLin/1 -> Sum/1
  VCirPt/1(vCir) -> Sum/2
  Demux/2 -> FxCir/1  "FxCir"
  wz/1 -> VCirPt/1(wz)
  Unit Vector/1 -> Components/1
  Sum/1 -> Friction Law/2
  Fn/1 -> Friction Law/1
  Line Ref h/1 -> TzLin/1
  Radius/1 -> TzCir/1
  Product2/1 -> Demux/1
  X Sep/1 -> Sign/1, VCirPt/2(X sep)
  Sign/1 -> Product1/2, Product3/2

== system Contact_Forces_Lib/2D/Circle to Ring Force/Forces/Ff/Resolve Ff ==
  note: Resolve Friction Force in
      | Circle B reference frame
      | Sign of Fn indicates
      | inside or outside ring.
  note: Resolve Friction Force in
      | Circle F reference frame
  Fn : Inport
  R : Inport  Port=2
  Ff : Inport  Port=3
  azm : Inport  Port=4
  Ff in CirB : Subsystem
  Ff in CirF : Subsystem
  Product : Product
  Sign : Signum  ZeroCross=off
  Tz : Subsystem
  FxCirF : Outport
  FyCirF : Outport  Port=2
  TzCirF : Outport  Port=3
  FxRinB : Outport  Port=4
  FyRinB : Outport  Port=5
  TzRinB : Outport  Port=6
  wires:
  Product/1 -> Ff in CirB/1(Ff)
  Sign/1 -> Product/2
  Fn/1 -> Sign/1
  Ff in CirF/1(FyCirF) -> FyCirF/1
  Ff in CirB/1(FxRinB) -> FxRinB/1, Ff in CirF/2(FxRinB)
  Ff in CirB/2(FyRinB) -> FyRinB/1, Ff in CirF/3(FyRinB)
  Ff in CirF/2(FxCirF) -> FxCirF/1
  Ff/1 -> Product/1, Tz/1(Ff)
  Tz/1(TzRinB) -> TzRinB/1
  Tz/2(TzCirF) -> TzCirF/1
  azm/1 -> Ff in CirB/2(azm)
  R/1 -> Ff in CirF/1(R)

== system Contact_Forces_Lib/2D/Circle to Ring Force/Forces/Ff/vTan ==
  Fn : Inport
  rad : Inport  Port=2
  Pen : Inport  Port=3
  vazm : Inport  Port=4
  wzf : Inport  Port=5
  Follower Radius : Constant  Value=radius_circle
  Midpt Pen : Gain  Gain=0.5
  Product1 : Product
  Product2 : Product
  Product3 : Product  Inputs=3
  Sign : Signum  ZeroCross=off
  Sum : Sum  Inputs=++-
  Sum1 : Sum  Inputs=+-
  Sum2 : Sum  Inputs=-+
  vTan : Outport
  wires:
  Sign/1 -> Product1/2, Product3/3
  Fn/1 -> Sign/1
  Product1/1 -> Sum/3
  Sum2/1 -> vTan/1
  Pen/1 -> Midpt Pen/1
  Sum/1 -> Product2/2
  rad/1 -> Sum/2
  Product2/1 -> Sum2/2  "vTan in B"
  Product3/1 -> Sum2/1  "vTan of F"
  Follower Radius/1 -> Sum1/1, Product1/1
  wzf/1 -> Product3/1
  vazm/1 -> Product2/1
  Midpt Pen/1 -> Sum1/2, Sum/1
  Sum1/1 -> Product3/2

== system Contact_Forces_Lib/2D/Circle to Ring Force/Forces/Fn/Fn in CirB ==
  Fn : Inport
  azm : Inport  Port=2
  Divide1 : Product  Inputs=**
  Divide2 : Product  Inputs=**
  Gain2 : Gain  Gain=-1
  cos : Trigonometry  Operator=cos
  deg2rad : Gain  Gain=pi/180
  sin : Trigonometry
  FxCirB : Outport
  FyCirB : Outport  Port=2
  wires:
  Gain2/1 -> Divide1/1, Divide2/1
  deg2rad/1 -> cos/1, sin/1
  sin/1 -> Divide2/2
  cos/1 -> Divide1/2
  Divide1/1 -> FxCirB/1
  Divide2/1 -> FyCirB/1
  Fn/1 -> Gain2/1
  azm/1 -> deg2rad/1

== system Contact_Forces_Lib/2D/Circle to Ring Force/Forces/Fn/Fn in CirF ==
  R : Inport
  FxCirB : Inport  Port=2
  FyCirB : Inport  Port=3
  Demux : Demux  Outputs=2
  Divide3 : Product  Inputs=**  Multiplication=Matrix(*)
  Gain : Gain  Gain=-1
  Mux1 : Mux  Inputs=2
  FyCirF : Outport
  FxCirF : Outport  Port=2
  wires:
  Demux/2 -> FxCirF/1
  Demux/1 -> FyCirF/1
  Gain/1 -> Demux/1
  Mux1/1 -> Divide3/2
  Divide3/1 -> Gain/1
  R/1 -> Divide3/1
  FyCirB/1 -> Mux1/1
  FxCirB/1 -> Mux1/2

== system Contact_Forces_Lib/2D/Composite Forces/Box to Belt Force/Belt Ends/Sensing C5 ==
  S : Inport
  Bus Selector : BusSelector  OutputSignals=Normal Force
  Fn : Outport
  wires:
  S/1 -> Bus Selector/1
  Bus Selector/1 -> Fn/1  "<Normal Force>"

== system Contact_Forces_Lib/2D/Composite Forces/Box to Belt Force/Belt Ends/Sensing C6 ==
  S : Inport
  Bus Selector : BusSelector  OutputSignals=Normal Force
  Fn : Outport
  wires:
  Bus Selector/1 -> Fn/1  "<Normal Force>"
  S/1 -> Bus Selector/1

== system Contact_Forces_Lib/2D/Composite Forces/Box to Belt Force/Belt Ends/Sensing C7 ==
  S : Inport
  Bus Selector : BusSelector  OutputSignals=Normal Force
  Fn : Outport
  wires:
  Bus Selector/1 -> Fn/1  "<Normal Force>"
  S/1 -> Bus Selector/1

== system Contact_Forces_Lib/2D/Composite Forces/Box to Belt Force/Belt Ends/Sensing C8 ==
  S : Inport
  Bus Selector : BusSelector  OutputSignals=Normal Force
  Fn : Outport
  wires:
  S/1 -> Bus Selector/1
  Bus Selector/1 -> Fn/1  "<Normal Force>"

== system Contact_Forces_Lib/2D/Composite Forces/Box to Belt Force/Belt Faces/Sensing C1 ==
  S : Inport
  Bus Selector : BusSelector  OutputSignals=Normal Force
  Fn : Outport
  wires:
  Bus Selector/1 -> Fn/1  "<Normal Force>"
  S/1 -> Bus Selector/1

== system Contact_Forces_Lib/2D/Composite Forces/Box to Belt Force/Belt Faces/Sensing C2 ==
  S : Inport
  Bus Selector : BusSelector  OutputSignals=Normal Force
  Fn : Outport
  wires:
  S/1 -> Bus Selector/1
  Bus Selector/1 -> Fn/1  "<Normal Force>"

== system Contact_Forces_Lib/2D/Composite Forces/Box to Belt Force/Belt Faces/Sensing C3 ==
  S : Inport
  Bus Selector : BusSelector  OutputSignals=Normal Force
  Fn : Outport
  wires:
  S/1 -> Bus Selector/1
  Bus Selector/1 -> Fn/1  "<Normal Force>"

== system Contact_Forces_Lib/2D/Composite Forces/Box to Belt Force/Belt Faces/Sensing C4 ==
  S : Inport
  Bus Selector : BusSelector  OutputSignals=Normal Force
  Fn : Outport
  wires:
  Bus Selector/1 -> Fn/1  "<Normal Force>"
  S/1 -> Bus Selector/1
